simulink model "Real_system_3_1_2"  (R2025b)
settings: Solver=ode5  StartTime=0.0  StopTime=45  FixedStep=0.001  RelTol=1e-3
undefined symbols (not defined in the file): Beq, degs2rpm, drv, gbox, Jeq, K_W, kd, ki, kp, mld, mot, National_Instruments, PCI, rdp, Req, sens, tl, Ts, u_bar_max
libraries: sldrtlib x3, simulink x1
settings Model: SimulationMode=external  ExtModeTrigDuration=45001  Creator=fasoloandr  LastModifiedBy=Enrico
settings DataIOCC: ReturnWorkspaceOutputsName=out_real_system
settings HardwareCC: ProdBitPerLong=64.0  ProdHWDeviceType=Intel->x86-64 (Linux 64)
settings RTWCC: SystemTargetFile=sldrt.tlc  TemplateMakefile=sldrt.tmf  RTWCompilerOptimization=on  Description=Simulink Desktop Real-Time
settings CodeAppCC: MaxIdLength=95.0
settings SimulinkDesktopRealTimeCC: ExtModeTransport=0.0  ExtModeStaticAllocSize=1000000.0  TargetLibSuffix=_sldrt.a  TargetPreCompLibLocation=D:\Programmi (D)\MATLAB\R2025b\toolbox\sldrt\lib\win64  MultiwordLength=2048.0  DynamicStringBufferSize=256.0  ParMdlRefBuildCompliant=on  PreserveMATLABNamespacesInGeneratedCode=on  SubcomponentCodeInterfacePackaging=Reusable function

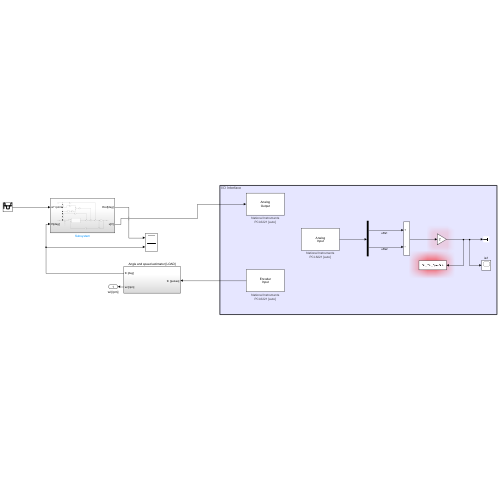
[thumbnail: Simulink's stored preview of the top-level diagram]
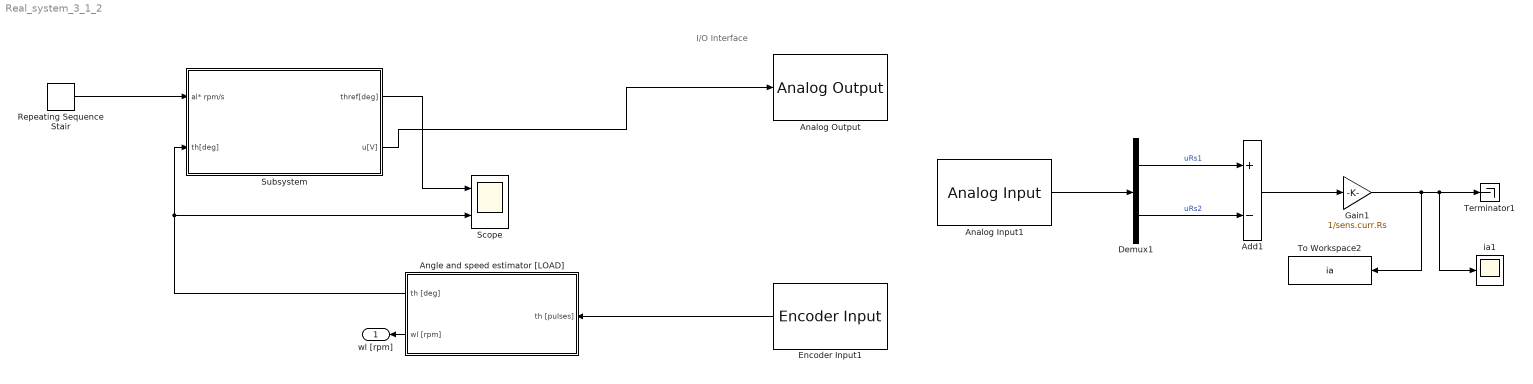
== system Real_system_3_1_2 ==
  note: I/O Interface
  Add1 : Sum  Inputs=+-
  Analog Input1 : sldrtlib/Analog Input  SampleTime=-1  MaxMissedTicks=10  ShowMissedTicks=off  YieldWhenWaiting=off  DrvName=National_Instruments/PCI-6221  DrvAddress=4294967295  DrvOptions=[0 0 0 2 0]  Channels=[1,2]  RangeMode=1  VoltRange=1  DataType=1
      settings: AttributesFormatString=National Instruments\nPCI-6221 [auto]
  Analog Output : sldrtlib/Analog Output  SampleTime=-1  MaxMissedTicks=10  ShowMissedTicks=off  YieldWhenWaiting=off  DrvName=National_Instruments/PCI-6221  DrvAddress=4294967295  DrvOptions=[0 0 0 2 0]  Channels=1  RangeMode=1  VoltRange=1  InitialValue=[0]  FinalValue=[0]
      settings: AttributesFormatString=National Instruments\nPCI-6221 [auto]
  Angle and speed estimator [LOAD] : Subsystem
  Demux1 : Demux  Outputs=2
  Encoder Input1 : sldrtlib/Encoder Input  SampleTime=-1  MaxMissedTicks=10  ShowMissedTicks=off  YieldWhenWaiting=off  DrvName=National_Instruments/PCI-6221  DrvAddress=4294967295  DrvOptions=[0 0 0 2 0]  Channels=1  QuadMode=3  IndexPulse=1  InputFilter=Inf  DataType=1
      settings: AttributesFormatString=National Instruments\nPCI-6221 [auto]
  Gain1 : Gain  Gain=1/sens.curr.Rs
  Repeating Sequence Stair : simulink/Sources/Repeating Sequence Stair  OutValues=[900 0 -900 -900 0 900]  tsamp=0.5  OutMin=[]  OutMax=[]  OutDataTypeStr=double  OutputDataTypeScalingMode=double  OutDataType=fixdt(0,8)  ConRadixGroup=Best Precision: Vector-wise  OutScaling=2^-12
  Scope : Scope  NumInputPorts=2
  Subsystem : Subsystem
  Terminator1 : Terminator
  To Workspace2 : ToWorkspace  VariableName=ia  SaveFormat=Timeseries  SampleTime=Ts
  ia1 : Scope
      settings: ActiveDisplayYMinimum=-1  ActiveDisplayYMaximum=1  DataLoggingVariableName=ScopeData2
  wl [rpm] : Outport
  wires:
  Add1/1 -> Gain1/1
  Demux1/1 -> Add1/1  "uRs1"
  Demux1/2 -> Add1/2  "uRs2"
  Gain1/1 -> To Workspace2/1, ia1/1, Terminator1/1
  Encoder Input1/1 -> Angle and speed estimator [LOAD]/1(th [pulses])
  Angle and speed estimator [LOAD]/1(th [deg]) -> Subsystem/2(th[deg]), Scope/2
  Angle and speed estimator [LOAD]/2(wl [rpm]) -> wl [rpm]/1
  Subsystem/2(u[V]) -> Analog Output/1
  Analog Input1/1 -> Demux1/1
  Repeating Sequence Stair/1 -> Subsystem/1(al* rpm/s)
  Subsystem/1(thref[deg]) -> Scope/1

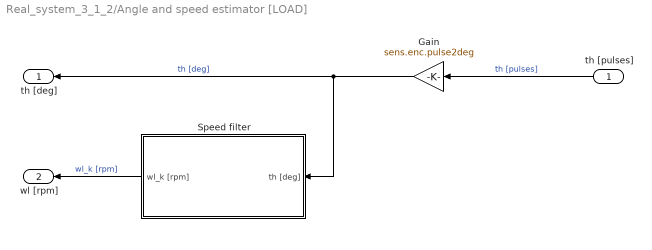
== system Real_system_3_1_2/Angle and speed estimator [LOAD] ==
  th [pulses] : Inport
  Gain : Gain  Gain=sens.enc.pulse2deg
  Speed filter : Subsystem
  th [deg] : Outport
  wl [rpm] : Outport  Port=2
  wires:
  Speed filter/1(wl_k [rpm]) -> wl [rpm]/1  "wl_k [rpm]"
  th [pulses]/1 -> Gain/1  "th [pulses]"
  Gain/1 -> Speed filter/1(th [deg]), th [deg]/1  "th [deg]"

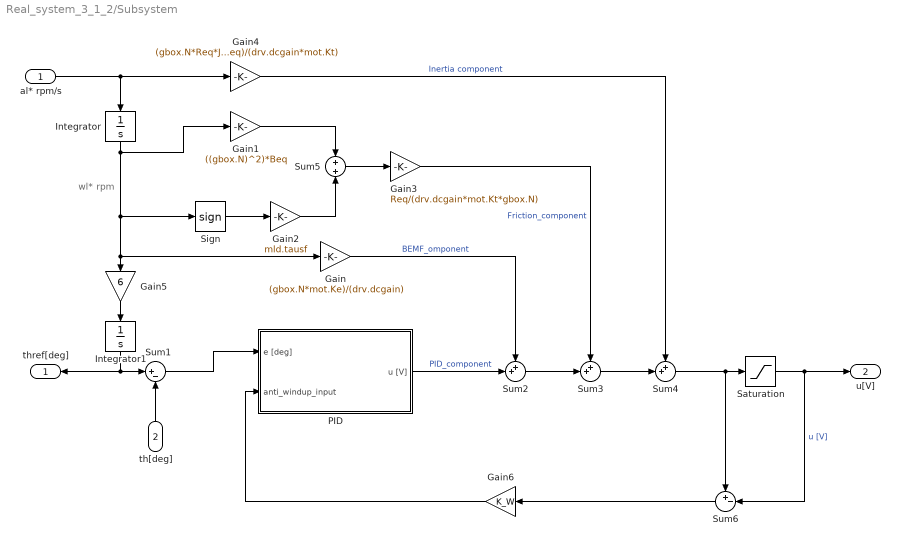
== system Real_system_3_1_2/Subsystem ==
  note: rpm
  note: wl*
  al* rpm/s : Inport
  th[deg] : Inport  Port=2
  Gain : Gain  Gain=(gbox.N*mot.Ke)/(drv.dcgain)
  Gain1 : Gain  Gain=((gbox.N)^2)*Beq
  Gain2 : Gain  Gain=mld.tausf
  Gain3 : Gain  Gain=Req/(drv.dcgain*mot.Kt*gbox.N)
  Gain4 : Gain  Gain=(gbox.N*Req*Jeq)/(drv.dcgain*mot.Kt)
  Gain5 : Gain  Gain=6
  Gain6 : Gain  Gain=K_W
  Integrator : Integrator
  Integrator1 : Integrator
  PID : Subsystem
  "Saturation " : Saturate  UpperLimit=u_bar_max  LowerLimit=-u_bar_max
  Sign : Signum
  Sum1 : Sum  Inputs=|+-
  Sum2 : Sum  Inputs=++|
  Sum3 : Sum  Inputs=++|
  Sum4 : Sum  Inputs=++|
  Sum5 : Sum  Inputs=+|+
  Sum6 : Sum  Inputs=+-|
  thref[deg] : Outport
  u[V] : Outport  Port=2
  wires:
  Sum3/1 -> Sum4/2
  Gain2/1 -> Sum5/2
  Integrator/1 -> Sign/1, Gain5/1, Gain/1, Gain1/1
  Sum2/1 -> Sum3/2
  Integrator1/1 -> thref[deg]/1, Sum1/1
  Gain3/1 -> Sum3/1  "Friction_component"
  PID/1(u [V]) -> Sum2/2  "PID_component"
  Sum5/1 -> Gain3/1
  Gain1/1 -> Sum5/1
  Gain5/1 -> Integrator1/1
  Sign/1 -> Gain2/1
  Sum1/1 -> PID/1(e [deg])
  Gain4/1 -> Sum4/1  "Inertia component"
  al* rpm/s/1 -> Gain4/1, Integrator/1
  th[deg]/1 -> Sum1/2
  Sum4/1 -> Sum6/1, "Saturation "/1
  "Saturation "/1 -> Sum6/2, u[V]/1  "u [V]"
  Sum6/1 -> Gain6/1
  Gain/1 -> Sum2/1  "BEMF_omponent"
  Gain6/1 -> PID/2(anti_windup_input)

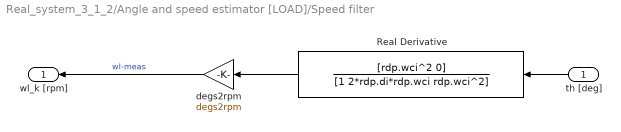
== system Real_system_3_1_2/Angle and speed estimator [LOAD]/Speed filter ==
  th [deg] : Inport
  Real Derivative : TransferFcn  Numerator=[rdp.wci^2 0]  Denominator=[1 2*rdp.di*rdp.wci rdp.wci^2]
  degs2rpm : Gain  Gain=degs2rpm
  wl_k [rpm] : Outport
  wires:
  th [deg]/1 -> Real Derivative/1
  degs2rpm/1 -> wl_k [rpm]/1  "wl-meas"
  Real Derivative/1 -> degs2rpm/1

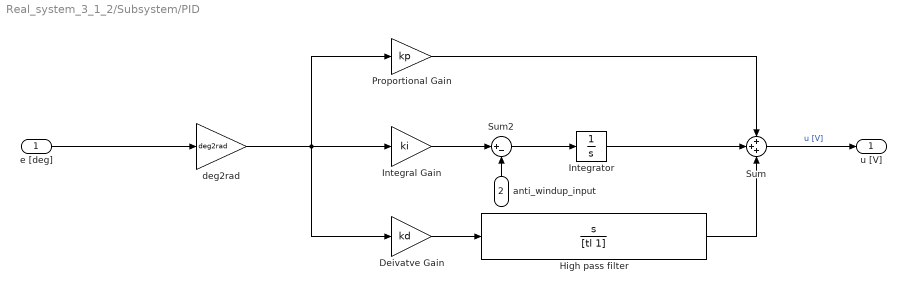
== system Real_system_3_1_2/Subsystem/PID ==
  e [deg] : Inport
  anti_windup_input : Inport  Port=2
  Deivatve Gain : Gain  Gain=kd
  High pass filter : TransferFcn  Numerator=[1 0]  Denominator=[tl 1]
  Integral Gain : Gain  Gain=ki
  Integrator : Integrator
  Proportional Gain : Gain  Gain=kp
  Sum : Sum  Inputs=+++
  Sum2 : Sum  Inputs=|+-
  deg2rad : Gain  Gain=deg2rad
  u [V] : Outport
  wires:
  Deivatve Gain/1 -> High pass filter/1
  e [deg]/1 -> deg2rad/1
  Integrator/1 -> Sum/2
  Sum/1 -> u [V]/1  "u [V]"
  deg2rad/1 -> Deivatve Gain/1, Proportional Gain/1, Integral Gain/1
  High pass filter/1 -> Sum/3
  Proportional Gain/1 -> Sum/1
  Sum2/1 -> Integrator/1
  Integral Gain/1 -> Sum2/1
  anti_windup_input/1 -> Sum2/2
